simulink model "a3_quan_control_differentialflatness"  (R2018b)
settings: Solver=VariableStepAuto  StartTime=0.0  StopTime=20  RelTol=1e-3
undefined symbols (not defined in the file or in its folder): AngularState, Attitude, AttitudeController, DifferentialFlat, drawQuad, InverseMapping, LQRController, P, PlotTrajectory, State, Trajectory
settings Model: Creator=erics  LastModifiedBy=erics

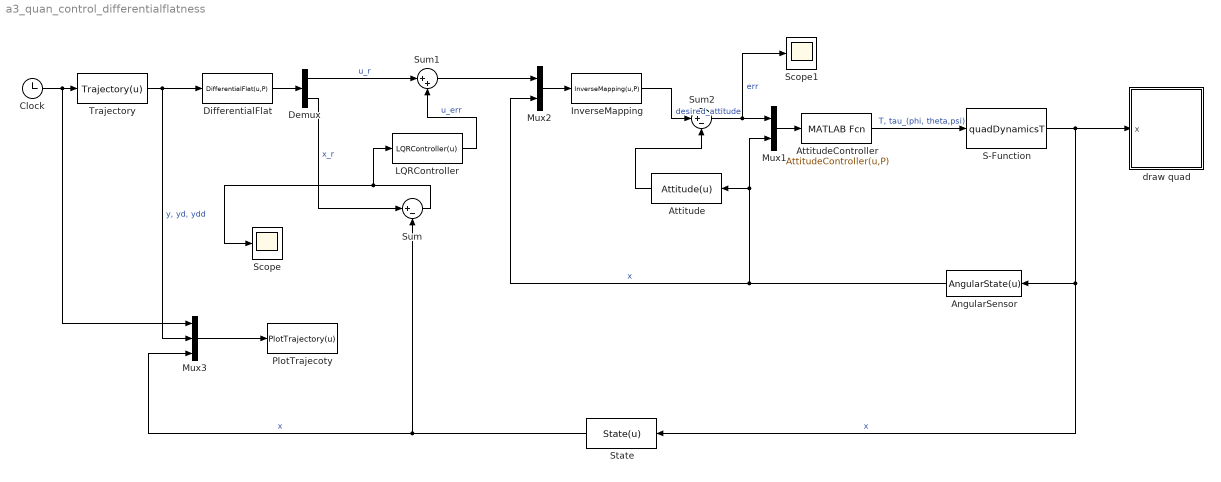
== system a3_quan_control_differentialflatness ==
  AngularSensor : MATLABFcn  MATLABFcn=AngularState(u)  OutputDimensions=6
  Attitude : MATLABFcn  MATLABFcn=Attitude(u)  OutputDimensions=4
  AttitudeController : MATLABFcn  MATLABFcn=AttitudeController(u,P)  OutputDimensions=4
  Clock : Clock
  Demux : Demux  Outputs=[4,-1]
  DifferentialFlat : MATLABFcn  MATLABFcn=DifferentialFlat(u,P)  OutputDimensions=11
  InverseMapping : MATLABFcn  MATLABFcn=InverseMapping(u,P)  OutputDimensions=4
  LQRController : MATLABFcn  MATLABFcn=LQRController(u)  OutputDimensions=4  Output1D=off
  Mux1 : Mux  Inputs=2
  Mux2 : Mux  Inputs=2
  Mux3 : Mux  Inputs=3
  PlotTrajecoty : MATLABFcn  MATLABFcn=PlotTrajectory(u)  OutputDimensions=0
  S-Function : S-Function  FunctionName=quadDynamicsT  Parameters=P  SFunctionDeploymentMode=off  EnableBusSupport=off
  Scope : Scope
  Scope1 : Scope
  State : MATLABFcn  MATLABFcn=State(u)  OutputDimensions=7
  Sum : Sum  Inputs=|+-
  Sum1 : Sum  Inputs=|++
  Sum2 : Sum  Inputs=|+-
  "Trajectory " : MATLABFcn  MATLABFcn=Trajectory(u)  OutputDimensions=12
  draw quad : Subsystem
      mask init:
      | P.courselength = 11;
      | P.coursewidth = 6;
      |     %6ft columns plus four feet of head room
      | P.courseheight = 10;
      | 
      | % quadrotor starting point at 3 ft high and 3 ft in front of the pillars 
      | P.zstart = 0;
      | P.xstart = 0;
      | P.ystart = 0;
      | 
      | % quadrotor dimentions
      |     %2 inches from the center
      | P.boxlength = 1/6;
      | P.boxwidth = P.boxlength;
      |     %4.5 inches from the bottom to the top
      | P.boxheight = 0.375;
      |     %6 inches from box to motor
      | P.armlength = 0.5;
      |     %1/8 inch from center to the side of a rod
      | P.armwidth = 1/96;
      |     %1/4 inch from the top of the box
      | P.armposition = 1/48;
      |     %25*(2)^(1/2)/2 inches from center to perimeter along x and y axis
      | P.perimeter = 1.47;
      |     %perimeter has 3/16 inch width
      | P.periwidth = 1/64;
      | 
      | % pillar dimentions
      |     %6 ft high
      | P.pillarheight = 6;
      |     %5 ft offset;
      | P.pillarposition = 5; 
      |     %5 in radius
      | P.pillarradius = 0.417;
      |     %The adjustment for the none circular pillar
      | P.pillaradd = 0.167;
      |     %The height of each strip on color
      | P.pillarc1 = 0.833; 
      | P.pillarc2 = 0.5;
      mask Display: image(imread('tv.jpg'))
  wires:
  S-Function/1 -> State/1, AngularSensor/1, draw quad/1(x)  "x"
  Clock/1 -> Mux3/1, "Trajectory "/1
  AttitudeController/1 -> S-Function/1  "T, tau_(phi, theta,psi)"
  Mux1/1 -> AttitudeController/1
  "Trajectory "/1 -> Mux3/2, DifferentialFlat/1  "y, yd, ydd"
  Mux2/1 -> InverseMapping/1
  DifferentialFlat/1 -> Demux/1
  Demux/2 -> Sum/1  "x_r"
  Sum/1 -> Scope/1, LQRController/1
  Demux/1 -> Sum1/1  "u_r"
  LQRController/1 -> Sum1/2  "u_err"
  Sum1/1 -> Mux2/1
  State/1 -> Sum/2, Mux3/3  "x"
  InverseMapping/1 -> Sum2/1  "desired_attitude"
  Attitude/1 -> Sum2/2
  Sum2/1 -> Scope1/1, Mux1/1  "err"
  Mux3/1 -> PlotTrajecoty/1
  AngularSensor/1 -> Attitude/1, Mux1/2, Mux2/2  "x"

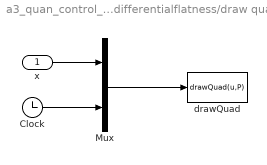
== system a3_quan_control_differentialflatness/draw quad ==
  x : Inport
  Clock : Clock
  Mux : Mux  Inputs=2
  drawQuad : MATLABFcn  MATLABFcn=drawQuad(u,P)  OutputDimensions=0  SampleTime=0.1
  wires:
  Mux/1 -> drawQuad/1
  x/1 -> Mux/1
  Clock/1 -> Mux/2
